simulink model "HMI_2L_StMdXX_Rsp"  (R2018b)
settings: Solver=FixedStepDiscrete  StartTime=0.0  StopTime=10.0  FixedStep=0.01  RelTol=1e-3
undefined symbols (not defined in the file or in its folder): KeSMSuRspStatHldTm_Val, SrcReqTp1
libraries: RspLib x20
(part 2 of 2)

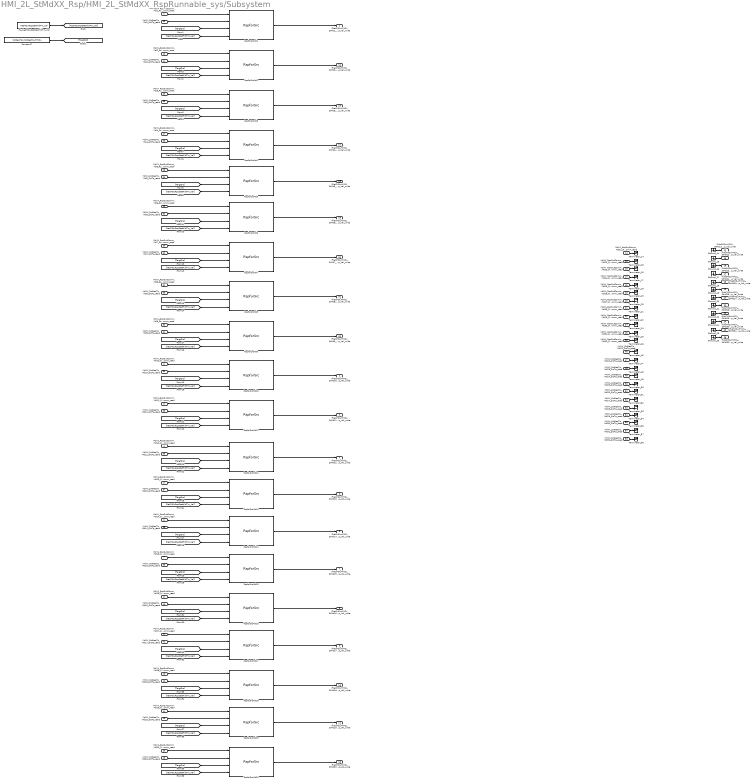
== system HMI_2L_StMdXX_Rsp/HMI_2L_StMdXX_RspRunnable_sys/Subsystem ==
  MdXX_RspOutComm_Md1_RspOutComm_read : Inport
  MdXX_RspOutComm_Md10_RspOutComm_read : Inport  Port=2
  MdXX_RspOutComm_Md11_RspOutComm_read : Inport  Port=3
  MdXX_RspOutComm_Md12_RspOutComm_read : Inport  Port=4
  MdXX_RspOutComm_Md13_RspOutComm_read : Inport  Port=5
  MdXX_RspOutComm_Md14_RspOutComm_read : Inport  Port=6
  MdXX_RspOutComm_Md15_RspOutComm_read : Inport  Port=7
  MdXX_RspOutComm_Md16_RspOutComm_read : Inport  Port=8
  MdXX_RspOutComm_Md17_RspOutComm_read : Inport  Port=9
  MdXX_RspOutComm_Md18_RspOutComm_read : Inport  Port=10
  MdXX_RspOutComm_Md19_RspOutComm_read : Inport  Port=11
  MdXX_RspOutComm_Md2_RspOutComm_read : Inport  Port=12
  MdXX_RspOutComm_Md20_RspOutComm_read : Inport  Port=13
  MdXX_RspOutComm_Md21_RspOutComm_read : Inport  Port=14
  MdXX_RspOutComm_Md22_RspOutComm_read : Inport  Port=15
  MdXX_RspOutComm_Md23_RspOutComm_read : Inport  Port=16
  MdXX_RspOutComm_Md24_RspOutComm_read : Inport  Port=17
  MdXX_RspOutComm_Md25_RspOutComm_read : Inport  Port=18
  MdXX_RspOutComm_Md26_RspOutComm_read : Inport  Port=19
  MdXX_RspOutComm_Md27_RspOutComm_read : Inport  Port=20
  MdXX_RspOutComm_Md28_RspOutComm_read : Inport  Port=21
  MdXX_RspOutComm_Md29_RspOutComm_read : Inport  Port=22
  MdXX_RspOutComm_Md3_RspOutComm_read : Inport  Port=23
  MdXX_RspOutComm_Md30_RspOutComm_read : Inport  Port=24
  MdXX_RspOutComm_Md31_RspOutComm_read : Inport  Port=25
  MdXX_RspOutComm_Md32_RspOutComm_read : Inport  Port=26
  MdXX_RspOutComm_Md4_RspOutComm_read : Inport  Port=27
  MdXX_RspOutComm_Md5_RspOutComm_read : Inport  Port=28
  MdXX_RspOutComm_Md6_RspOutComm_read : Inport  Port=29
  MdXX_RspOutComm_Md7_RspOutComm_read : Inport  Port=30
  MdXX_RspOutComm_Md8_RspOutComm_read : Inport  Port=31
  MdXX_RspOutComm_Md9_RspOutComm_read : Inport  Port=32
  MdXX_SrcReqTp_Md1_SrcTp_read : Inport  Port=33
  MdXX_SrcReqTp_Md10_SrcTp_read : Inport  Port=34
  MdXX_SrcReqTp_Md11_SrcTp_read : Inport  Port=35
  MdXX_SrcReqTp_Md12_SrcTp_read : Inport  Port=36
  MdXX_SrcReqTp_Md13_SrcTp_read : Inport  Port=37
  MdXX_SrcReqTp_Md14_SrcTp_read : Inport  Port=38
  MdXX_SrcReqTp_Md15_SrcTp_read : Inport  Port=39
  MdXX_SrcReqTp_Md16_SrcTp_read : Inport  Port=40
  MdXX_SrcReqTp_Md17_SrcTp_read : Inport  Port=41
  MdXX_SrcReqTp_Md18_SrcTp_read : Inport  Port=42
  MdXX_SrcReqTp_Md19_SrcTp_read : Inport  Port=43
  MdXX_SrcReqTp_Md2_SrcTp_read : Inport  Port=44
  MdXX_SrcReqTp_Md20_SrcTp_read : Inport  Port=45
  MdXX_SrcReqTp_Md21_SrcTp_read : Inport  Port=46
  MdXX_SrcReqTp_Md22_SrcTp_read : Inport  Port=47
  MdXX_SrcReqTp_Md23_SrcTp_read : Inport  Port=48
  MdXX_SrcReqTp_Md24_SrcTp_read : Inport  Port=49
  MdXX_SrcReqTp_Md25_SrcTp_read : Inport  Port=50
  MdXX_SrcReqTp_Md26_SrcTp_read : Inport  Port=51
  MdXX_SrcReqTp_Md27_SrcTp_read : Inport  Port=52
  MdXX_SrcReqTp_Md28_SrcTp_read : Inport  Port=53
  MdXX_SrcReqTp_Md29_SrcTp_read : Inport  Port=54
  MdXX_SrcReqTp_Md3_SrcTp_read : Inport  Port=55
  MdXX_SrcReqTp_Md30_SrcTp_read : Inport  Port=56
  MdXX_SrcReqTp_Md31_SrcTp_read : Inport  Port=57
  MdXX_SrcReqTp_Md32_SrcTp_read : Inport  Port=58
  MdXX_SrcReqTp_Md4_SrcTp_read : Inport  Port=59
  MdXX_SrcReqTp_Md5_SrcTp_read : Inport  Port=60
  MdXX_SrcReqTp_Md6_SrcTp_read : Inport  Port=61
  MdXX_SrcReqTp_Md7_SrcTp_read : Inport  Port=62
  MdXX_SrcReqTp_Md8_SrcTp_read : Inport  Port=63
  MdXX_SrcReqTp_Md9_SrcTp_read : Inport  Port=64
  Constant7 : Constant  Value=SrcReqTp1.SrcReqTp_HMI2L  OutDataTypeStr=Enum:SrcReqTp1
  Ground_{14..22,24..26} (12 alike) : Ground
  PA_KeSMSuRspStatHldTm_Val : Constant  Value=KeSMSuRspStatHldTm_Val
  RspforSrcMd{1..20} (20 alike) : RspLib/RspforSrc  SystemSampleTime=-1
  Terminator_{14..22,24..26,46..54,56..58} (24 alike) : Terminator
  IfVeSMSuHMI2L_StMd1_Rsp_Val_write : Outport
      settings: EnsureOutportIsVirtual=on
  IfVeSMSuHMI2L_StMd10_Rsp_Val_write : Outport  Port=2
      settings: EnsureOutportIsVirtual=on
  IfVeSMSuHMI2L_StMd11_Rsp_Val_write : Outport  Port=3
      settings: EnsureOutportIsVirtual=on
  IfVeSMSuHMI2L_StMd12_Rsp_Val_write : Outport  Port=4
      settings: EnsureOutportIsVirtual=on
  IfVeSMSuHMI2L_StMd13_Rsp_Val_write : Outport  Port=5
      settings: EnsureOutportIsVirtual=on
  IfVeSMSuHMI2L_StMd14_Rsp_Val_write : Outport  Port=6
      settings: EnsureOutportIsVirtual=on
  IfVeSMSuHMI2L_StMd15_Rsp_Val_write : Outport  Port=7
      settings: EnsureOutportIsVirtual=on
  IfVeSMSuHMI2L_StMd16_Rsp_Val_write : Outport  Port=8
      settings: EnsureOutportIsVirtual=on
  IfVeSMSuHMI2L_StMd17_Rsp_Val_write : Outport  Port=9
      settings: EnsureOutportIsVirtual=on
  IfVeSMSuHMI2L_StMd18_Rsp_Val_write : Outport  Port=10
      settings: EnsureOutportIsVirtual=on
  IfVeSMSuHMI2L_StMd19_Rsp_Val_write : Outport  Port=11
      settings: EnsureOutportIsVirtual=on
  IfVeSMSuHMI2L_StMd2_Rsp_Val_write : Outport  Port=12
      settings: EnsureOutportIsVirtual=on
  IfVeSMSuHMI2L_StMd20_Rsp_Val_write : Outport  Port=13
      settings: EnsureOutportIsVirtual=on
  IfVeSMSuHMI2L_StMd21_Rsp_Val_write : Outport  Port=14
      settings: EnsureOutportIsVirtual=on
  IfVeSMSuHMI2L_StMd22_Rsp_Val_write : Outport  Port=15
      settings: EnsureOutportIsVirtual=on
  IfVeSMSuHMI2L_StMd23_Rsp_Val_write : Outport  Port=16
      settings: EnsureOutportIsVirtual=on
  IfVeSMSuHMI2L_StMd24_Rsp_Val_write : Outport  Port=17
      settings: EnsureOutportIsVirtual=on
  IfVeSMSuHMI2L_StMd25_Rsp_Val_write : Outport  Port=18
      settings: EnsureOutportIsVirtual=on
  IfVeSMSuHMI2L_StMd26_Rsp_Val_write : Outport  Port=19
      settings: EnsureOutportIsVirtual=on
  IfVeSMSuHMI2L_StMd27_Rsp_Val_write : Outport  Port=20
      settings: EnsureOutportIsVirtual=on
  IfVeSMSuHMI2L_StMd28_Rsp_Val_write : Outport  Port=21
      settings: EnsureOutportIsVirtual=on
  IfVeSMSuHMI2L_StMd29_Rsp_Val_write : Outport  Port=22
      settings: EnsureOutportIsVirtual=on
  IfVeSMSuHMI2L_StMd3_Rsp_Val_write : Outport  Port=23
      settings: EnsureOutportIsVirtual=on
  IfVeSMSuHMI2L_StMd30_Rsp_Val_write : Outport  Port=24
      settings: EnsureOutportIsVirtual=on
  IfVeSMSuHMI2L_StMd31_Rsp_Val_write : Outport  Port=25
      settings: EnsureOutportIsVirtual=on
  IfVeSMSuHMI2L_StMd32_Rsp_Val_write : Outport  Port=26
      settings: EnsureOutportIsVirtual=on
  IfVeSMSuHMI2L_StMd4_Rsp_Val_write : Outport  Port=27
      settings: EnsureOutportIsVirtual=on
  IfVeSMSuHMI2L_StMd5_Rsp_Val_write : Outport  Port=28
      settings: EnsureOutportIsVirtual=on
  IfVeSMSuHMI2L_StMd6_Rsp_Val_write : Outport  Port=29
      settings: EnsureOutportIsVirtual=on
  IfVeSMSuHMI2L_StMd7_Rsp_Val_write : Outport  Port=30
      settings: EnsureOutportIsVirtual=on
  IfVeSMSuHMI2L_StMd8_Rsp_Val_write : Outport  Port=31
      settings: EnsureOutportIsVirtual=on
  IfVeSMSuHMI2L_StMd9_Rsp_Val_write : Outport  Port=32
      settings: EnsureOutportIsVirtual=on
  wires:
  MdXX_RspOutComm_Md32_RspOutComm_read/1 -> Terminator_26/1
  MdXX_RspOutComm_Md26_RspOutComm_read/1 -> Terminator_19/1
  MdXX_SrcReqTp_Md28_SrcTp_read/1 -> Terminator_53/1
  MdXX_RspOutComm_Md30_RspOutComm_read/1 -> Terminator_24/1
  MdXX_SrcReqTp_Md29_SrcTp_read/1 -> Terminator_54/1
  MdXX_RspOutComm_Md22_RspOutComm_read/1 -> Terminator_15/1
  MdXX_RspOutComm_Md28_RspOutComm_read/1 -> Terminator_21/1
  MdXX_RspOutComm_Md23_RspOutComm_read/1 -> Terminator_16/1
  Ground_24/1 -> IfVeSMSuHMI2L_StMd30_Rsp_Val_write/1
  MdXX_RspOutComm_Md25_RspOutComm_read/1 -> Terminator_18/1
  PA_KeSMSuRspStatHldTm_Val/1 -> [KeSMSuRspStatHldTm_Val]
  MdXX_SrcReqTp_Md21_SrcTp_read/1 -> Terminator_46/1
  MdXX_RspOutComm_Md31_RspOutComm_read/1 -> Terminator_25/1
  MdXX_RspOutComm_Md29_RspOutComm_read/1 -> Terminator_22/1
  MdXX_SrcReqTp_Md23_SrcTp_read/1 -> Terminator_48/1
  MdXX_SrcReqTp_Md22_SrcTp_read/1 -> Terminator_47/1
  MdXX_RspOutComm_Md21_RspOutComm_read/1 -> Terminator_14/1
  MdXX_SrcReqTp_Md26_SrcTp_read/1 -> Terminator_51/1
  Ground_17/1 -> IfVeSMSuHMI2L_StMd24_Rsp_Val_write/1
  Ground_16/1 -> IfVeSMSuHMI2L_StMd23_Rsp_Val_write/1
  MdXX_SrcReqTp_Md30_SrcTp_read/1 -> Terminator_56/1
  MdXX_SrcReqTp_Md24_SrcTp_read/1 -> Terminator_49/1
  MdXX_SrcReqTp_Md25_SrcTp_read/1 -> Terminator_50/1
  Ground_18/1 -> IfVeSMSuHMI2L_StMd25_Rsp_Val_write/1
  MdXX_RspOutComm_Md24_RspOutComm_read/1 -> Terminator_17/1
  MdXX_RspOutComm_Md27_RspOutComm_read/1 -> Terminator_20/1
  Ground_14/1 -> IfVeSMSuHMI2L_StMd21_Rsp_Val_write/1
  Ground_20/1 -> IfVeSMSuHMI2L_StMd27_Rsp_Val_write/1
  Ground_26/1 -> IfVeSMSuHMI2L_StMd32_Rsp_Val_write/1
  Ground_25/1 -> IfVeSMSuHMI2L_StMd31_Rsp_Val_write/1
  MdXX_SrcReqTp_Md31_SrcTp_read/1 -> Terminator_57/1
  Ground_19/1 -> IfVeSMSuHMI2L_StMd26_Rsp_Val_write/1
  MdXX_SrcReqTp_Md32_SrcTp_read/1 -> Terminator_58/1
  Ground_22/1 -> IfVeSMSuHMI2L_StMd29_Rsp_Val_write/1
  MdXX_SrcReqTp_Md27_SrcTp_read/1 -> Terminator_52/1
  Ground_21/1 -> IfVeSMSuHMI2L_StMd28_Rsp_Val_write/1
  Ground_15/1 -> IfVeSMSuHMI2L_StMd22_Rsp_Val_write/1
  MdXX_RspOutComm_Md1_RspOutComm_read/1 -> RspforSrcMd1/1
  [KeSMSuRspStatHldTm_Val] -> RspforSrcMd1/4
  Constant7/1 -> [TargtSrc]
  [TargtSrc] -> RspforSrcMd1/3
  MdXX_SrcReqTp_Md1_SrcTp_read/1 -> RspforSrcMd1/2
  RspforSrcMd1/1 -> IfVeSMSuHMI2L_StMd1_Rsp_Val_write/1
  RspforSrcMd2/1 -> IfVeSMSuHMI2L_StMd2_Rsp_Val_write/1
  MdXX_SrcReqTp_Md2_SrcTp_read/1 -> RspforSrcMd2/2
  [TargtSrc] -> RspforSrcMd2/3
  [KeSMSuRspStatHldTm_Val] -> RspforSrcMd2/4
  MdXX_RspOutComm_Md2_RspOutComm_read/1 -> RspforSrcMd2/1
  MdXX_RspOutComm_Md3_RspOutComm_read/1 -> RspforSrcMd3/1
  [KeSMSuRspStatHldTm_Val] -> RspforSrcMd3/4
  [TargtSrc] -> RspforSrcMd3/3
  MdXX_SrcReqTp_Md3_SrcTp_read/1 -> RspforSrcMd3/2
  RspforSrcMd3/1 -> IfVeSMSuHMI2L_StMd3_Rsp_Val_write/1
  RspforSrcMd4/1 -> IfVeSMSuHMI2L_StMd4_Rsp_Val_write/1
  MdXX_SrcReqTp_Md4_SrcTp_read/1 -> RspforSrcMd4/2
  [TargtSrc] -> RspforSrcMd4/3
  [KeSMSuRspStatHldTm_Val] -> RspforSrcMd4/4
  MdXX_RspOutComm_Md4_RspOutComm_read/1 -> RspforSrcMd4/1
  MdXX_RspOutComm_Md5_RspOutComm_read/1 -> RspforSrcMd5/1
  [KeSMSuRspStatHldTm_Val] -> RspforSrcMd5/4
  [TargtSrc] -> RspforSrcMd5/3
  MdXX_SrcReqTp_Md5_SrcTp_read/1 -> RspforSrcMd5/2
  RspforSrcMd5/1 -> IfVeSMSuHMI2L_StMd5_Rsp_Val_write/1
  RspforSrcMd6/1 -> IfVeSMSuHMI2L_StMd6_Rsp_Val_write/1
  MdXX_SrcReqTp_Md6_SrcTp_read/1 -> RspforSrcMd6/2
  [TargtSrc] -> RspforSrcMd6/3
  [KeSMSuRspStatHldTm_Val] -> RspforSrcMd6/4
  MdXX_RspOutComm_Md6_RspOutComm_read/1 -> RspforSrcMd6/1
  MdXX_RspOutComm_Md7_RspOutComm_read/1 -> RspforSrcMd7/1
  [KeSMSuRspStatHldTm_Val] -> RspforSrcMd7/4
  [TargtSrc] -> RspforSrcMd7/3
  MdXX_SrcReqTp_Md7_SrcTp_read/1 -> RspforSrcMd7/2
  RspforSrcMd7/1 -> IfVeSMSuHMI2L_StMd7_Rsp_Val_write/1
  RspforSrcMd8/1 -> IfVeSMSuHMI2L_StMd8_Rsp_Val_write/1
  MdXX_SrcReqTp_Md8_SrcTp_read/1 -> RspforSrcMd8/2
  [TargtSrc] -> RspforSrcMd8/3
  [KeSMSuRspStatHldTm_Val] -> RspforSrcMd8/4
  MdXX_RspOutComm_Md8_RspOutComm_read/1 -> RspforSrcMd8/1
  MdXX_RspOutComm_Md9_RspOutComm_read/1 -> RspforSrcMd9/1
  [KeSMSuRspStatHldTm_Val] -> RspforSrcMd9/4
  [TargtSrc] -> RspforSrcMd9/3
  MdXX_SrcReqTp_Md9_SrcTp_read/1 -> RspforSrcMd9/2
  RspforSrcMd9/1 -> IfVeSMSuHMI2L_StMd9_Rsp_Val_write/1
  RspforSrcMd10/1 -> IfVeSMSuHMI2L_StMd10_Rsp_Val_write/1
  MdXX_SrcReqTp_Md10_SrcTp_read/1 -> RspforSrcMd10/2
  [TargtSrc] -> RspforSrcMd10/3
  [KeSMSuRspStatHldTm_Val] -> RspforSrcMd10/4
  MdXX_RspOutComm_Md10_RspOutComm_read/1 -> RspforSrcMd10/1
  MdXX_RspOutComm_Md11_RspOutComm_read/1 -> RspforSrcMd11/1
  [KeSMSuRspStatHldTm_Val] -> RspforSrcMd11/4
  [TargtSrc] -> RspforSrcMd11/3
  MdXX_SrcReqTp_Md11_SrcTp_read/1 -> RspforSrcMd11/2
  RspforSrcMd11/1 -> IfVeSMSuHMI2L_StMd11_Rsp_Val_write/1
  RspforSrcMd12/1 -> IfVeSMSuHMI2L_StMd12_Rsp_Val_write/1
  MdXX_SrcReqTp_Md12_SrcTp_read/1 -> RspforSrcMd12/2
  [TargtSrc] -> RspforSrcMd12/3
  [KeSMSuRspStatHldTm_Val] -> RspforSrcMd12/4
  MdXX_RspOutComm_Md12_RspOutComm_read/1 -> RspforSrcMd12/1
  MdXX_RspOutComm_Md13_RspOutComm_read/1 -> RspforSrcMd13/1
  [KeSMSuRspStatHldTm_Val] -> RspforSrcMd13/4
  [TargtSrc] -> RspforSrcMd13/3
  MdXX_SrcReqTp_Md13_SrcTp_read/1 -> RspforSrcMd13/2
  RspforSrcMd13/1 -> IfVeSMSuHMI2L_StMd13_Rsp_Val_write/1
  RspforSrcMd14/1 -> IfVeSMSuHMI2L_StMd14_Rsp_Val_write/1
  MdXX_SrcReqTp_Md14_SrcTp_read/1 -> RspforSrcMd14/2
  [TargtSrc] -> RspforSrcMd14/3
  [KeSMSuRspStatHldTm_Val] -> RspforSrcMd14/4
  MdXX_RspOutComm_Md14_RspOutComm_read/1 -> RspforSrcMd14/1
  MdXX_RspOutComm_Md15_RspOutComm_read/1 -> RspforSrcMd15/1
  [KeSMSuRspStatHldTm_Val] -> RspforSrcMd15/4
  [TargtSrc] -> RspforSrcMd15/3
  MdXX_SrcReqTp_Md15_SrcTp_read/1 -> RspforSrcMd15/2
  RspforSrcMd15/1 -> IfVeSMSuHMI2L_StMd15_Rsp_Val_write/1
  RspforSrcMd16/1 -> IfVeSMSuHMI2L_StMd16_Rsp_Val_write/1
  MdXX_SrcReqTp_Md16_SrcTp_read/1 -> RspforSrcMd16/2
  [TargtSrc] -> RspforSrcMd16/3
  [KeSMSuRspStatHldTm_Val] -> RspforSrcMd16/4
  MdXX_RspOutComm_Md16_RspOutComm_read/1 -> RspforSrcMd16/1
  MdXX_RspOutComm_Md17_RspOutComm_read/1 -> RspforSrcMd17/1
  [KeSMSuRspStatHldTm_Val] -> RspforSrcMd17/4
  [TargtSrc] -> RspforSrcMd17/3
  MdXX_SrcReqTp_Md17_SrcTp_read/1 -> RspforSrcMd17/2
  RspforSrcMd17/1 -> IfVeSMSuHMI2L_StMd17_Rsp_Val_write/1
  RspforSrcMd18/1 -> IfVeSMSuHMI2L_StMd18_Rsp_Val_write/1
  MdXX_SrcReqTp_Md18_SrcTp_read/1 -> RspforSrcMd18/2
  [TargtSrc] -> RspforSrcMd18/3
  [KeSMSuRspStatHldTm_Val] -> RspforSrcMd18/4
  MdXX_RspOutComm_Md18_RspOutComm_read/1 -> RspforSrcMd18/1
  MdXX_RspOutComm_Md19_RspOutComm_read/1 -> RspforSrcMd19/1
  [KeSMSuRspStatHldTm_Val] -> RspforSrcMd19/4
  [TargtSrc] -> RspforSrcMd19/3
  MdXX_SrcReqTp_Md19_SrcTp_read/1 -> RspforSrcMd19/2
  RspforSrcMd19/1 -> IfVeSMSuHMI2L_StMd19_Rsp_Val_write/1
  RspforSrcMd20/1 -> IfVeSMSuHMI2L_StMd20_Rsp_Val_write/1
  MdXX_SrcReqTp_Md20_SrcTp_read/1 -> RspforSrcMd20/2
  [TargtSrc] -> RspforSrcMd20/3
  [KeSMSuRspStatHldTm_Val] -> RspforSrcMd20/4
  MdXX_RspOutComm_Md20_RspOutComm_read/1 -> RspforSrcMd20/1
